simulink model "observer"  (R2022b)
settings: Solver=VariableStepAuto  StartTime=0.0  StopTime=30  RelTol=1e-3
values from neighbouring files (symbols this model uses):
  Cd = ss_d.C    [lab12.m]
  Dd = ss_d.D    [lab12.m]
  disturbio = 0.24    [lab12.m]
  F = ss_d.A    [lab12.m]
  H = ss_d.B    [lab12.m]
  L = Lt'    [lab12.m]
  R = 1.18    [lab12.m]
  sistema_inicial = [-0.11; -0.11]    [lab12.m]
  T0 = 0.203    [lab12.m]
settings Model: Creator=mathe  LastModifiedBy=mathe

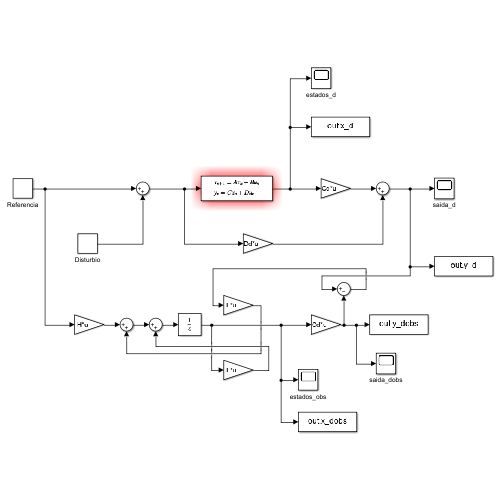
[thumbnail: Simulink's stored preview of the top-level diagram]
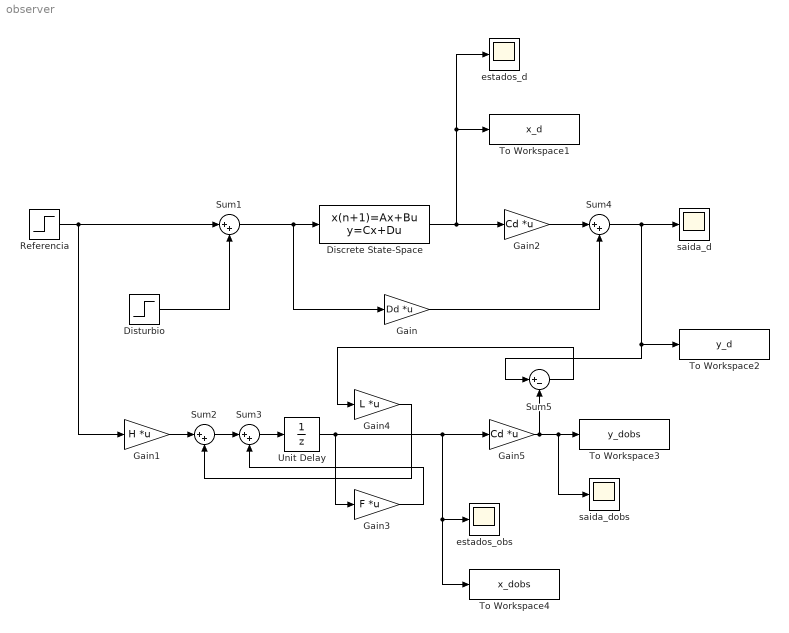
== system observer ==
  Discrete State-Space : DiscreteStateSpace  A=F  B=H  C=[1 0; 0 1]  D=[0; 0]  InitialCondition=sistema_inicial  SampleTime=T0
  Disturbio : Step  Time=15  After=disturbio  SampleTime=0
  Gain : Gain  Gain=Dd  Multiplication=Matrix(K*u)
  Gain1 : Gain  Gain=H  Multiplication=Matrix(K*u)
  Gain2 : Gain  Gain=Cd  Multiplication=Matrix(K*u)
  Gain3 : Gain  Gain=F  Multiplication=Matrix(K*u)
  Gain4 : Gain  Gain=L  Multiplication=Matrix(K*u)
  Gain5 : Gain  Gain=Cd  Multiplication=Matrix(K*u)
  Referencia : Step  Time=0  After=R  SampleTime=0
  Sum{1..4} (4 alike) : Sum  Inputs=|++
  Sum5 : Sum  Inputs=|+-
  To Workspace1 : ToWorkspace  VariableName=x_d  SaveFormat=Timeseries  SampleTime=-1
  To Workspace2 : ToWorkspace  VariableName=y_d  SaveFormat=Timeseries  SampleTime=-1
  To Workspace3 : ToWorkspace  VariableName=y_dobs  SaveFormat=Timeseries  SampleTime=-1
  To Workspace4 : ToWorkspace  VariableName=x_dobs  SaveFormat=Timeseries  SampleTime=-1
  Unit Delay : UnitDelay  SampleTime=-1  HasFrameUpgradeWarning=on
  estados_d : Scope
  estados_obs : Scope
  saida_d : Scope
  saida_dobs : Scope
  wires:
  Discrete State-Space/1 -> Gain2/1, estados_d/1, To Workspace1/1
  Sum4/1 -> Sum5/1, To Workspace2/1, saida_d/1
  Sum1/1 -> Discrete State-Space/1, Gain/1
  Referencia/1 -> Gain1/1, Sum1/1
  Disturbio/1 -> Sum1/2
  Gain2/1 -> Sum4/1
  Gain/1 -> Sum4/2
  Gain1/1 -> Sum2/1
  Sum2/1 -> Sum3/1
  Gain3/1 -> Sum3/2
  Gain4/1 -> Sum2/2
  Gain5/1 -> Sum5/2, saida_dobs/1, To Workspace3/1
  Sum3/1 -> Unit Delay/1
  Unit Delay/1 -> Gain3/1, To Workspace4/1, estados_obs/1, Gain5/1
  Sum5/1 -> Gain4/1
